simulink library "EV3Fcns"  (R2014b)
settings: Solver=ode45  StartTime=0.0  StopTime=10.0  RelTol=1e-3
libraries: legoev3lib x3, legonxtlib x2
settings Model: Creator=pvinnako  LastModifiedBy=pkaniara

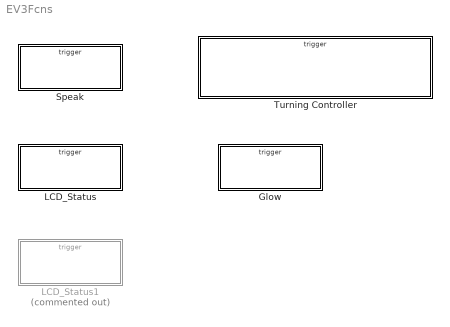
== system EV3Fcns ==
  Glow : Subsystem  AncestorBlock=EV3Fcns/Speak  TreatAsAtomicUnit=on
  LCD_Status : Subsystem  TreatAsAtomicUnit=on
  LCD_Status1 : Subsystem  Commented=on  TreatAsAtomicUnit=on
  Speak : Subsystem  TreatAsAtomicUnit=on
  Turning Controller : Subsystem  AncestorBlock=SimControllerFcns/Turning Controller  TreatAsAtomicUnit=on

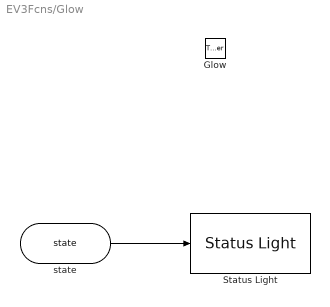
== system EV3Fcns/Glow ==
  Glow : TriggerPort  TriggerType=function-call  IsSimulinkFunction=on  FunctionName=Glow
  Status Light : legoev3lib/Status Light
  state : ArgIn  ArgumentName=state
  wires:
  state/1 -> Status Light/1

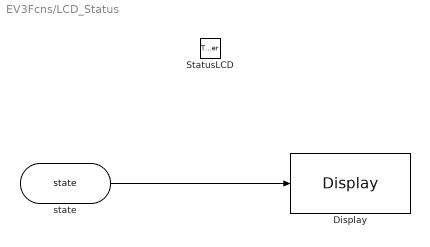
== system EV3Fcns/LCD_Status ==
  StatusLCD : TriggerPort  TriggerType=function-call  IsSimulinkFunction=on  FunctionName=StatusLCD
  Display : legoev3lib/Display  slcdStr=state  slcdLine=10  slcdFormat=Decimal
  state : ArgIn  ArgumentName=state
  wires:
  state/1 -> Display/1

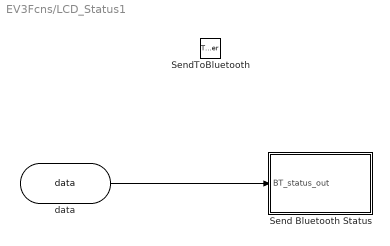
== system EV3Fcns/LCD_Status1 ==
  SendToBluetooth : TriggerPort  TriggerType=function-call  IsSimulinkFunction=on  FunctionName=SendToBluetooth
  Send Bluetooth Status : Subsystem  Variant=on  OverrideUsingVariant=BluetoothOFF
  data : ArgIn  OutDataTypeStr=uint16  ArgumentName=data
  wires:
  data/1 -> Send Bluetooth Status/1(BT_status_out)

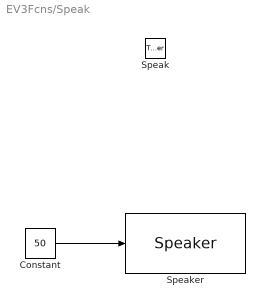
== system EV3Fcns/Speak ==
  Speak : TriggerPort  TriggerType=function-call  IsSimulinkFunction=on  FunctionName=Speak
  Constant : Constant  Value=50
  Speaker : legoev3lib/Speaker  sinputMode=Volume only  sspeakerFreq=100  sspeakerVolume=50  sspeakerDuration=100
  wires:
  Constant/1 -> Speaker/1

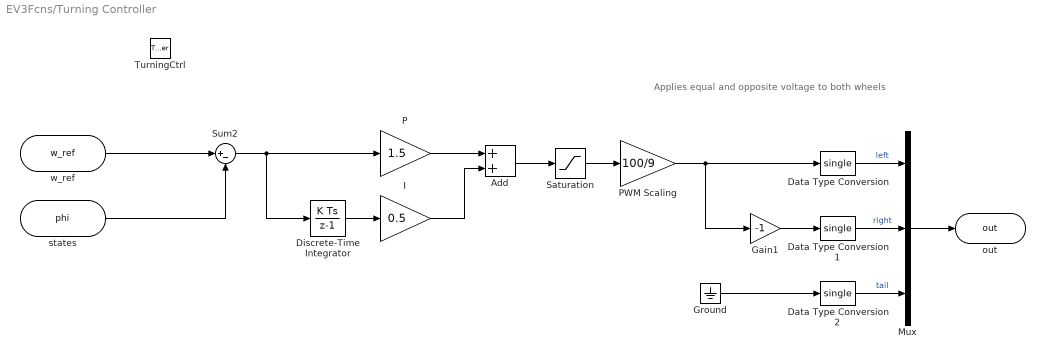
== system EV3Fcns/Turning Controller ==
  note: Applies equal and opposite voltage to both wheels
  TurningCtrl : TriggerPort  TriggerType=function-call  IsSimulinkFunction=on  FunctionName=TurningCtrl
  Add : Sum
  Data Type Conversion : DataTypeConversion  OutDataTypeStr=single
  Data Type Conversion1 : DataTypeConversion  OutDataTypeStr=single
  Data Type Conversion2 : DataTypeConversion  OutDataTypeStr=single
  Discrete-Time Integrator : DiscreteIntegrator  SampleTime=-1
  Gain1 : Gain  Gain=-1
  Ground : Ground
  I : Gain  Gain=0.5
  Mux : Mux  Inputs=3
  P : Gain  Gain=1.5
  PWM Scaling : Gain  Gain=100/9
  Saturation : Saturate  UpperLimit=2  LowerLimit=-2
  Sum2 : Sum  Inputs=|+-
  w_ref : ArgIn  OutDataTypeStr=single  ArgumentName=w_ref
  states : ArgIn  Port=2  OutDataTypeStr=single  ArgumentName=phi
  out : ArgOut  OutDataTypeStr=single  PortDimensions=3  ArgumentName=out
  wires:
  Data Type Conversion2/1 -> Mux/3  "tail"
  Data Type Conversion1/1 -> Mux/2  "right"
  Data Type Conversion/1 -> Mux/1  "left"
  Ground/1 -> Data Type Conversion2/1
  P/1 -> Add/1
  states/1 -> Sum2/2
  Sum2/1 -> Discrete-Time Integrator/1, P/1
  PWM Scaling/1 -> Data Type Conversion/1, Gain1/1
  w_ref/1 -> Sum2/1
  Mux/1 -> out/1
  Add/1 -> Saturation/1
  I/1 -> Add/2
  Discrete-Time Integrator/1 -> I/1
  Saturation/1 -> PWM Scaling/1
  Gain1/1 -> Data Type Conversion1/1

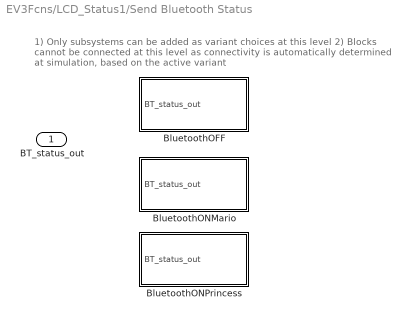
== system EV3Fcns/LCD_Status1/Send Bluetooth Status ==
  note: 1) Only subsystems can be added as variant choices at this level
      | 2) Blocks cannot be connected at this level as connectivity is
      | automatically determined at simulation, based on the active variant
  BT_status_out : Inport
  BluetoothOFF : Subsystem  VariantControl=BluetoothOFF
  BluetoothONMario : Subsystem  VariantControl=BluetoothONMario
  BluetoothONPrincess : Subsystem  VariantControl=BluetoothONPrincess

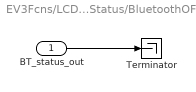
== system EV3Fcns/LCD_Status1/Send Bluetooth Status/BluetoothOFF ==
  BT_status_out : Inport
  Terminator : Terminator
  wires:
  BT_status_out/1 -> Terminator/1

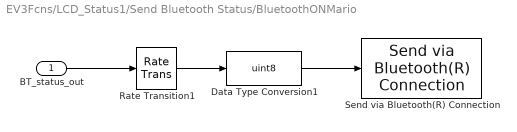
== system EV3Fcns/LCD_Status1/Send Bluetooth Status/BluetoothONMario ==
  BT_status_out : Inport
  Data Type Conversion1 : DataTypeConversion  OutDataTypeStr=uint8
  Rate Transition1 : RateTransition  OutPortSampleTime=0.1
  Send via Bluetooth(R) Connection : legonxtlib/Send via Bluetooth(R) Connection  mailbox=4
  wires:
  BT_status_out/1 -> Rate Transition1/1
  Rate Transition1/1 -> Data Type Conversion1/1
  Data Type Conversion1/1 -> Send via Bluetooth(R) Connection/1

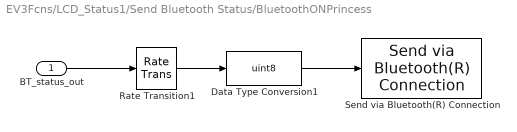
== system EV3Fcns/LCD_Status1/Send Bluetooth Status/BluetoothONPrincess ==
  BT_status_out : Inport
  Data Type Conversion1 : DataTypeConversion  OutDataTypeStr=uint8
  Rate Transition1 : RateTransition  OutPortSampleTime=0.1
  Send via Bluetooth(R) Connection : legonxtlib/Send via Bluetooth(R) Connection  mailbox=3
  wires:
  Data Type Conversion1/1 -> Send via Bluetooth(R) Connection/1
  Rate Transition1/1 -> Data Type Conversion1/1
  BT_status_out/1 -> Rate Transition1/1
